simulink model "control_algorithm_models"  (R2016a)
settings: Solver=ode4  StartTime=0.0  StopTime=Tfinal  FixedStep=Ts  RelTol=1e-3
values from neighbouring files (symbols this model uses):
  Ef = 155    [control_simulation_parameters.m]    (also in pmsm_vbyf_sim_parameters.m = 80)
  fout = 100    [control_simulation_parameters.m]    (also in pmsm_vbyf_sim_parameters.m; vbyfcontrolim_sim.m = 50)
  fsw = 10e3    (= 10000)    [control_simulation_parameters.m]    (also in pmsm_vbyf_sim_parameters.m; vbyfcontrolim_sim.m)
  Ki = 100    [control_simulation_parameters.m]
  Kp = 100    [control_simulation_parameters.m]
  motor_speed = 600    [control_simulation_parameters.m]
  pole_pair = 10    [control_simulation_parameters.m]    (also in pmsm_vbyf_sim_parameters.m)
  Ts = 1e-6    (= 1e-06)    [control_simulation_parameters.m]    (also in pmsm_vbyf_sim_parameters.m; vbyfcontrolim_sim.m)
  Tsw = 1/fsw    (= 0.0001)    [control_simulation_parameters.m]    (also in vbyfcontrolim_sim.m)
  Ymax = 300    [control_simulation_parameters.m]
  Ymin = -300    [control_simulation_parameters.m]
libraries: powerlib x9, powerlib_meascontrol x8, simulink x2
settings Model: Creator=ugurm  LastModifiedBy=mesutto
settings DataIOCC: LimitDataPoints=on  SaveFormat=Array
settings DebuggingCC: UnderspecifiedInitializationDetection=Classic  MergeDetectMultiDrivingBlocksExec=none  SolverPrmCheckMsg=warning  StateNameClashWarn=warning
settings HardwareCC: ProdBitPerPointer=32  ProdLargestAtomicFloat=None  ProdIntDivRoundTo=Undefined  ProdEndianess=Unspecified  ProdWordSize=32  ProdHWDeviceType=32-bit Generic
settings ModelReferenceCC: PropagateSignalLabelsOutOfModel=off
settings ConfigComp: CovModelRefEnable=Off

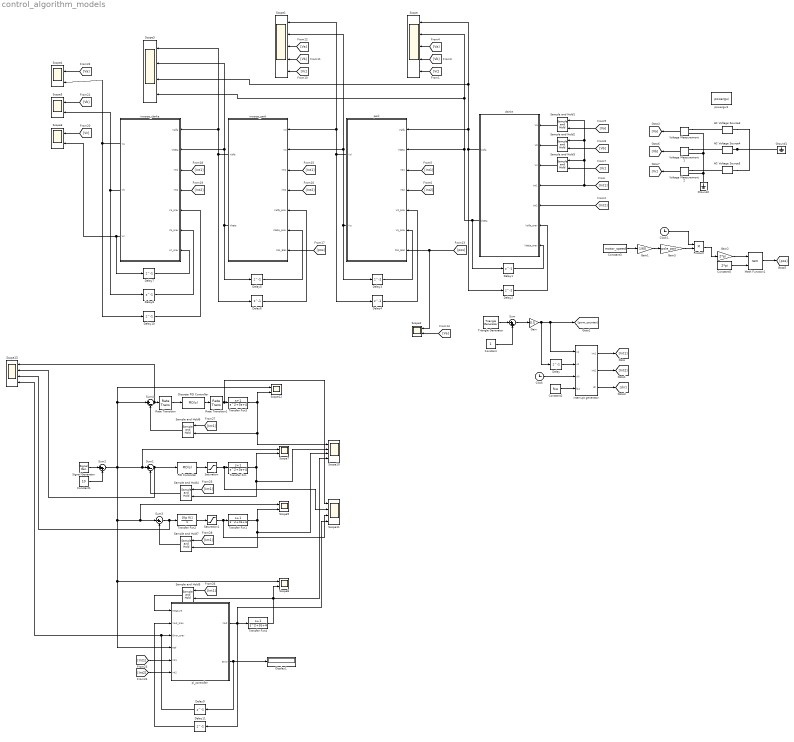
== system control_algorithm_models ==
  AC Voltage Source3 : powerlib/Electrical Sources/AC Voltage Source  Amplitude=Ef*sqrt(2)  Phase=0  Frequency=fout  SampleTime=0  Measurements=None  BusType=swing  Pref=10e3  Qref=0  Qmin=-inf  Qmax=+inf
  AC Voltage Source4 : powerlib/Electrical Sources/AC Voltage Source  Amplitude=Ef*sqrt(2)  Phase=-120  Frequency=fout  SampleTime=0  Measurements=None  BusType=swing  Pref=10e3  Qref=0  Qmin=-inf  Qmax=+inf
  AC Voltage Source5 : powerlib/Electrical Sources/AC Voltage Source  Amplitude=Ef*sqrt(2)  Phase=-240  Frequency=fout  SampleTime=0  Measurements=None  BusType=swing  Pref=10e3  Qref=0  Qmin=-inf  Qmax=+inf
  Clock : Clock
  Clock1 : Clock
  Constant : Constant
  Constant1 : Constant  Value=10
  Constant2 : Constant  Value=fsw
  Constant3 : Constant  Value=motor_speed
  Constant5 : Constant  Value=2*pi
  Delay{,1..11} (12 alike) : Delay  DelayLength=1
  Discrete PID Controller : simulink/Continuous/PID Controller  Controller=PID  TimeDomain=Discrete-time  SampleTime=Tsw  IntegratorMethod=Forward Euler  FilterMethod=Forward Euler  Form=Parallel  UseFilter=on  ControllerParametersSource=internal  P=Kp  I=Ki  D=0  N=100  InitialConditionSource=internal  InitialConditionForIntegrator=0  InitialConditionForFilter=0  ExternalReset=none  LimitOutput=on  UpperSaturationLimit=Ymax  LowerSaturationLimit=Ymin  LinearizeAsGain=off  AntiWindupMode=none  Kb=1  TrackingMode=off  Kt=1  PParamMin=[]  PParamMax=[]  IParamMin=[]  IParamMax=[]  DParamMin=[]  DParamMax=[]  NParamMin=[]  NParamMax=[]  KbParamMin=[]  KbParamMax=[]  KtParamMin=[]  KtParamMax=[]  POutMin=[]  POutMax=[]  IOutMin=[]  IOutMax=[]  DOutMin=[]  DOutMax=[]  NOutMin=[]  NOutMax=[]  KbOutMin=[]  KbOutMax=[]  KtOutMin=[]  KtOutMax=[]  IntegratorOutMin=[]  IntegratorOutMax=[]  FilterOutMin=[]  FilterOutMax=[]  SumOutMin=[]  SumOutMax=[]  SumI1OutMin=[]  SumI1OutMax=[]  SumI2OutMin=[]  SumI2OutMax=[]  SumI3OutMin=[]  SumI3OutMax=[]  SumDOutMin=[]  SumDOutMax=[]  SaturationOutMin=[]  SaturationOutMax=[]  IntegratorContinuousStateAttributes=''  IntegratorStateMustResolveToSignalObject=off  IntegratorRTWStateStorageClass=Auto  FilterContinuousStateAttributes=''  FilterStateMustResolveToSignalObject=off  FilterRTWStateStorageClass=Auto  DifferentiatorICPrevScaledInput=0  DifferentiatorOutMin=[]  DifferentiatorOutMax=[]
  Display1 : Display
  Gain : Gain  Gain=0.5
  Gain1 : Gain  Gain=1/60
  Gain2 : Gain  Gain=2*pi
  Gain3 : Gain  Gain=pole_pair
  Ground1 : powerlib/Elements/Ground  LConnTagsString=a
  Ground2 : powerlib/Elements/Ground  LConnTagsString=a
  Math Function1 : Math  Operator=rem  SaturateOnIntegerOverflow=on
  PID Controller : simulink/Continuous/PID Controller  Controller=PID  TimeDomain=Continuous-time  SampleTime=-1  IntegratorMethod=Forward Euler  FilterMethod=Forward Euler  Form=Parallel  UseFilter=on  ControllerParametersSource=internal  P=Kp  I=Ki  D=0  N=100  InitialConditionSource=internal  InitialConditionForIntegrator=0  InitialConditionForFilter=0  ExternalReset=none  LimitOutput=off  UpperSaturationLimit=inf  LowerSaturationLimit=-inf  LinearizeAsGain=on  AntiWindupMode=none  Kb=1  TrackingMode=off  Kt=1  PParamMin=[]  PParamMax=[]  IParamMin=[]  IParamMax=[]  DParamMin=[]  DParamMax=[]  NParamMin=[]  NParamMax=[]  KbParamMin=[]  KbParamMax=[]  KtParamMin=[]  KtParamMax=[]  POutMin=[]  POutMax=[]  IOutMin=[]  IOutMax=[]  DOutMin=[]  DOutMax=[]  NOutMin=[]  NOutMax=[]  KbOutMin=[]  KbOutMax=[]  KtOutMin=[]  KtOutMax=[]  IntegratorOutMin=[]  IntegratorOutMax=[]  FilterOutMin=[]  FilterOutMax=[]  SumOutMin=[]  SumOutMax=[]  SumI1OutMin=[]  SumI1OutMax=[]  SumI2OutMin=[]  SumI2OutMax=[]  SumI3OutMin=[]  SumI3OutMax=[]  SumDOutMin=[]  SumDOutMax=[]  SaturationOutMin=[]  SaturationOutMax=[]  IntegratorContinuousStateAttributes=''  IntegratorStateMustResolveToSignalObject=off  IntegratorRTWStateStorageClass=Auto  FilterContinuousStateAttributes=''  FilterStateMustResolveToSignalObject=off  FilterRTWStateStorageClass=Auto  DifferentiatorICPrevScaledInput=0  DifferentiatorOutMin=[]  DifferentiatorOutMax=[]
  Product : Product
  Rate Transition : RateTransition  OutPortSampleTime=Tsw
  Rate Transition1 : RateTransition  OutPortSampleTime=Ts
  Sample and Hold{1..7} (7 alike) : powerlib_meascontrol/Additional Components/Sample and Hold  ic=0  Ts=0
  Saturation : Saturate  UpperLimit=Ymax  LowerLimit=Ymin
  Saturation1 : Saturate  UpperLimit=Ymax  LowerLimit=Ymin
  Scope : Scope  NumInputPorts=5
  Scope1 : Scope  NumInputPorts=5
  Scope{3,10..11,13} (4 alike) : Scope  NumInputPorts=4
  Scope{2,4..9,12} (8 alike) : Scope  NumInputPorts=2
  Signal Generator : SignalGenerator  WaveForm=square  Amplitude=5  Frequency=2
  Sum : Sum  Inputs=|++
  Sum1 : Sum  Inputs=|+-
  Sum2 : Sum  Inputs=|++
  Sum3 : Sum  Inputs=|+-
  Sum4 : Sum  Inputs=|+-
  Transfer Fcn{,1,3..4} (4 alike) : TransferFcn  Numerator=[1 1]  Denominator=[1 3 4]
  Transfer Fcn2 : TransferFcn  Numerator=[Kp Ki]  Denominator=[1 0]
  Triangle Generator : powerlib_meascontrol/Pulse & Signal Generators/Triangle Generator  Freq=fsw  Phase=0  Ts=Ts
  Voltage Measurement : powerlib/Measurements/Voltage Measurement  PhasorSimulation=off  OutputType=Complex  PSBequivalent=0
  Voltage Measurement1 : powerlib/Measurements/Voltage Measurement  PhasorSimulation=off  OutputType=Complex  PSBequivalent=0
  Voltage Measurement2 : powerlib/Measurements/Voltage Measurement  PhasorSimulation=off  OutputType=Complex  PSBequivalent=0
  clarke : MATLAB Function  TreatAsAtomicUnit=on
  interrupt generator : MATLAB Function  TreatAsAtomicUnit=on
  inverse_clarke : MATLAB Function  TreatAsAtomicUnit=on
  inverse_park : MATLAB Function  TreatAsAtomicUnit=on
  park : MATLAB Function  TreatAsAtomicUnit=on
  pi_controller : MATLAB Function  TreatAsAtomicUnit=on
  powergui1 : powerlib/powergui  Priority=1  SimulationMode=Discrete  SolverType=Tustin  SampleTime=Ts  frequency=60  SPID=off  DisableSnubberDevices=off  DisableRonSwitches=off  DisableVfSwitches=off  SwTol=0  DisplayEquations=off  Interpol=off  ExternalGateDelay=off  methode=off  Ts=0  FunctionMessages=off  echomessages=off  HookPort=off  EnableUseOfTLC=off  x0status=blocks  frequencyindice=100  Pbase=100e6  ErrMax=1e-4  Iterations=50  UnitsV=kV  UnitsW=MW  buscounter=0  RestoreLinks=warning  ResistiveCurrentMeasurement=off  Frange=[0:2:500]  Ylog=off  Xlog=on  ShowGrid=off  save=off  variable=ZData  structure=Vdc  ZoomFFT=on  StartTime=0.04  cycles=5  DisplayStyle=5  fundamental=50  FreqAxis=off  MaxFrequency=30000  frequencyindicesteady=1  RmsSteady=1  display=off
  wires:
  Triangle Generator/1 -> Sum/1
  Constant/1 -> Sum/2
  Sum/1 -> Gain/1
  Gain/1 -> [pwm_counter], interrupt generator/1(u1), Delay/1
  Delay/1 -> interrupt generator/2(u2)
  Clock/1 -> interrupt generator/3(clk)
  Constant2/1 -> interrupt generator/4(fsw)
  interrupt generator/1(int1) -> [Int1]
  interrupt generator/2(int2) -> [Int2]
  interrupt generator/3(dir) -> [dir]
  [Va] -> Sample and Hold1/1
  [Vb] -> Sample and Hold2/1
  [Vc] -> Sample and Hold3/1
  Voltage Measurement/1 -> [Va]
  Voltage Measurement1/1 -> [Vb]
  Voltage Measurement2/1 -> [Vc]
  [Int1] -> clarke/4(int1), Sample and Hold3/2, Sample and Hold2/2, Sample and Hold1/2
  [Int2] -> clarke/5(int2)
  Sample and Hold1/1 -> clarke/1(Va)
  Sample and Hold2/1 -> clarke/2(Vb)
  Sample and Hold3/1 -> clarke/3(Vc)
  Delay1/1 -> clarke/7(Vbeta_prev)
  Delay2/1 -> clarke/6(Valfa_prev)
  [Va] -> Scope/3
  [Vb] -> Scope/4
  [Vc] -> Scope/5
  [Int2] -> park/4(int2)
  [Int1] -> park/3(int1)
  Delay3/1 -> park/6(Vq_prev)
  Delay4/1 -> park/5(Vd_prev)
  park/1(Vd) -> inverse_park/1(Vd), Scope1/1, Delay4/1
  park/2(Vq) -> Delay3/1, inverse_park/2(Vq), Scope1/2
  [Va] -> Scope1/3
  [Vb] -> Scope1/4
  [Vc] -> Scope1/5
  Constant3/1 -> Gain1/1
  Gain1/1 -> Gain3/1
  Clock1/1 -> Product/1
  Product/1 -> Gain2/1
  Gain2/1 -> Math Function1/1
  Constant5/1 -> Math Function1/2
  Math Function1/1 -> [pos]
  [pos] -> Scope2/1, park/7(Pos_Elec)
  [Va] -> Scope2/2
  Gain3/1 -> Product/2
  [Int2] -> inverse_park/4(int2)
  [Int1] -> inverse_park/3(int1)
  Delay5/1 -> inverse_park/6(Vbeta_prev)
  inverse_park/2(Vbeta) -> Delay5/1, inverse_clarke/2(Vbeta), Scope3/2
  inverse_park/1(Valfa) -> Delay6/1, inverse_clarke/1(Valfa), Scope3/1
  Delay6/1 -> inverse_park/5(Valfa_prev)
  [pos] -> inverse_park/7(Pos_Elec)
  clarke/1(Valfa) -> Scope3/3, Scope/1, park/1(Valfa), Delay2/1
  clarke/2(Vbeta) -> Delay1/1, Scope3/4, Scope/2, park/2(Vbeta)
  [Int1] -> inverse_clarke/3(int1)
  [Int2] -> inverse_clarke/4(int2)
  Delay7/1 -> inverse_clarke/7(Vc_prev)
  Delay8/1 -> inverse_clarke/6(Vb_prev)
  Delay10/1 -> inverse_clarke/5(Va_prev)
  inverse_clarke/2(Vb) -> Delay8/1, Scope5/2
  [Va] -> Scope4/1
  [Vb] -> Scope5/1
  [Vc] -> Scope6/1
  inverse_clarke/1(Va) -> Delay10/1, Scope4/2
  inverse_clarke/3(Vc) -> Scope6/2, Delay7/1
  Sum1/1 -> PID Controller/1, Scope13/2
  Sum2/1 -> Scope9/1, Sum3/1, Scope8/1, pi_controller/4(Ref), Scope12/1, Sum4/1, Scope7/1, Sum1/1
  Transfer Fcn/1 -> Scope7/2, Sample and Hold4/1, Scope10/2
  PID Controller/1 -> Saturation/1
  Saturation/1 -> Scope11/2, Transfer Fcn/1
  Constant1/1 -> Sum2/2
  Signal Generator/1 -> Sum2/1
  pi_controller/2(Error) -> Display1/1, Delay9/1
  pi_controller/1(Yout) -> Scope11/4, Delay11/1, Transfer Fcn4/1
  Delay11/1 -> pi_controller/2(Yout_prev)
  Transfer Fcn4/1 -> Scope8/2, Scope10/4, Sample and Hold5/1
  [Int1] -> pi_controller/5(int1)
  [Int2] -> pi_controller/6(int2)
  Transfer Fcn2/1 -> Saturation1/1
  Sum3/1 -> Scope13/3, Transfer Fcn2/1
  Saturation1/1 -> Scope11/3, Transfer Fcn1/1
  Transfer Fcn1/1 -> Scope10/3, Sample and Hold7/1, Scope9/2
  Sample and Hold4/1 -> Sum1/2
  [Int1] -> Sample and Hold4/2
  Sample and Hold5/1 -> pi_controller/1(Measure)
  [Int1] -> Sample and Hold5/2
  Discrete PID Controller/1 -> Rate Transition1/1
  Sum4/1 -> Scope13/1, Rate Transition/1
  Transfer Fcn3/1 -> Scope10/1, Sample and Hold6/1, Scope12/2
  Sample and Hold6/1 -> Sum4/2
  [Int1] -> Sample and Hold6/2
  [Int1] -> Sample and Hold7/2
  Sample and Hold7/1 -> Sum3/2
  Rate Transition/1 -> Discrete PID Controller/1
  Rate Transition1/1 -> Scope11/1, Transfer Fcn3/1
  Delay9/1 -> Scope13/4, pi_controller/3(Error_prev)
  connections:
  AC Voltage Source4/LConn1 -- Ground1/LConn1 -- AC Voltage Source3/LConn1 -- AC Voltage Source5/LConn1
  Voltage Measurement/LConn1 -- AC Voltage Source3/RConn1
  Voltage Measurement2/LConn1 -- AC Voltage Source5/RConn1
  Voltage Measurement1/LConn1 -- AC Voltage Source4/RConn1
  Ground2/LConn1 -- Voltage Measurement/LConn2 -- Voltage Measurement1/LConn2 -- Voltage Measurement2/LConn2

== matlab function control_algorithm_models/clarke ==
  data: Va input; Valfa output; Vb input; Vc input; Vbeta output; int1 input; int2 input; Valfa_prev input; Vbeta_prev input
function [Valfa,Vbeta] = fcn(Va,Vb,Vc,int1,int2,Valfa_prev,Vbeta_prev)

if (int1 == 1) % interrupt on zero event
    
    % clarke transform for currents
    Valfa = (2/3)*Va - (1/3)*(Vb + Vc);
    Vbeta = (1/sqrt(3))*(Vb - Vc);
    
else
    Valfa = Valfa_prev;
    Vbeta = Vbeta_prev;
    
end;

if (int2 == 1) % interrupt on prd event
    
    
else
    
    
end;

== matlab function control_algorithm_models/park ==
  data: Valfa input; Vd output; Vbeta input; int1 input; int2 input; Vd_prev input; Vq output; Vq_prev input; Pos_Elec input
function [Vd,Vq] = fcn(Valfa,Vbeta,int1,int2,Vd_prev,Vq_prev,Pos_Elec)

if (int1 == 1) % interrupt on zero event
    
    % clarke transform for currents
    Vd = Valfa*cos(Pos_Elec) + Vbeta*sin(Pos_Elec);
    Vq = Valfa*sin(Pos_Elec) - Vbeta*cos(Pos_Elec);
    
else
    Vd = Vd_prev;
    Vq = Vq_prev;
    
end;

if (int2 == 1) % interrupt on prd event
    
    
else
    
    
end;

== matlab function control_algorithm_models/interrupt generator ==
  data: u1 input; int1 output; u2 input; clk input; int2 output; dir output; fsw input
function [int1,int2,dir] = fcn(u1,u2,clk,fsw)

if (rem(clk,1/fsw) == 0)
    int1 = 1; % interrupt on zero
    dir = 0;
else
    int1 = 0;
    if (u1 > u2)
        dir = 1; % up
    else
        dir = 0; % down
    end;
end;

if (rem(clk*2,1/fsw) == 0 && rem(clk,1/fsw) ~= 0)
    int2 = 1; % interrupt on period
else
    int2 = 0;
end;

== matlab function control_algorithm_models/inverse_park ==
  data: Vd input; Valfa output; Vq input; int1 input; int2 input; Valfa_prev input; Vbeta_prev input; Pos_Elec input; Vbeta output
function [Valfa,Vbeta] = fcn(Vd,Vq,int1,int2,Valfa_prev,Vbeta_prev,Pos_Elec)

if (int1 == 1) % interrupt on zero event
    
    Valfa = Vd*cos(Pos_Elec) + Vq*sin(Pos_Elec);   
    Vbeta = -Vq*cos(Pos_Elec) + Vd*sin(Pos_Elec);   
    
else
    Valfa = Valfa_prev;
    Vbeta = Vbeta_prev;
    
end;

if (int2 == 1) % interrupt on prd event
    
    
else
    
    
end;

== matlab function control_algorithm_models/inverse_clarke ==
  data: Valfa input; Va output; Vbeta input; int1 input; int2 input; Va_prev input; Vb_prev input; Vc_prev input; Vb output; Vc output
function [Va,Vb,Vc] = fcn(Valfa,Vbeta,int1,int2,Va_prev,Vb_prev,Vc_prev)

if (int1 == 1) % interrupt on zero event
    
    Va = Valfa;
    Vb = (-Valfa + sqrt(3)*Vbeta)/2;
    Vc = (-Valfa - sqrt(3)*Vbeta)/2;
    
else
    Va = Va_prev;
    Vb = Vb_prev;
    Vc = Vc_prev;
    
end;

if (int2 == 1) % interrupt on prd event
    
    
else
    
    
end;

== matlab function control_algorithm_models/pi_controller ==
  data: Measure input; Yout output; Yout_prev input; Error_prev input; Ref input; Error output; int1 input; int2 input
function [Yout,Error] = fcn(Measure,Yout_prev,Error_prev,Ref,int1,int2)
if (int1 == 1) % interrupt on zero event
    
    Kp = 100;
    Ki = 0.5;
    Ts = 1;
    %Ts = 1/10000;
    Ymax = 300;
    Ymin = -300;
    Error = Ref - Measure;
    Yout = Yout_prev + Error*(Kp+Ki) - Error_prev*(Kp);
    %Yout = Yout_prev + Error*(Kp+Ki*Ts/2) - Error_prev*(Kp-Ki*Ts/2);
    %Yout = Yout_prev + Error*(Kp) - Error_prev*(Kp-Ki*Ts);
    if (Yout > Ymax)
        Yout = Ymax;
    elseif (Yout < Ymin)
        Yout = Ymin;
    end
    
else
    Yout = Yout_prev;
    Error = Error_prev;
    
end;

if (int2 == 1) % interrupt on prd event
    
    
else
    
    
end;
